simulink model "Reaction_Wheel_Model"  (R2025a)
settings: Solver=VariableStepAuto  StartTime=0.0  StopTime=120  RelTol=1e-3
values from neighbouring files (symbols this model uses):
  J = Jm + Jdisk    (= 1.0323014)    [Reaction_Wheel_Model_Variables.m]
  Js = 0.0022    [Reaction_Wheel_Model_Variables.m]
  K = 0.022    [Reaction_Wheel_Model_Variables.m]
  L = 580*10^-6    (= 0.00058)    [Reaction_Wheel_Model_Variables.m]
  R = 5.3    [Reaction_Wheel_Model_Variables.m]
libraries: simulink_extras x2
settings Model: Creator=Stefan1  LastModifiedBy=Stefan1

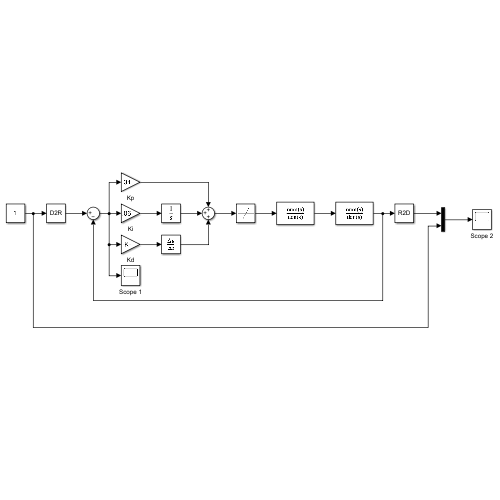
[thumbnail: Simulink's stored preview of the top-level diagram]
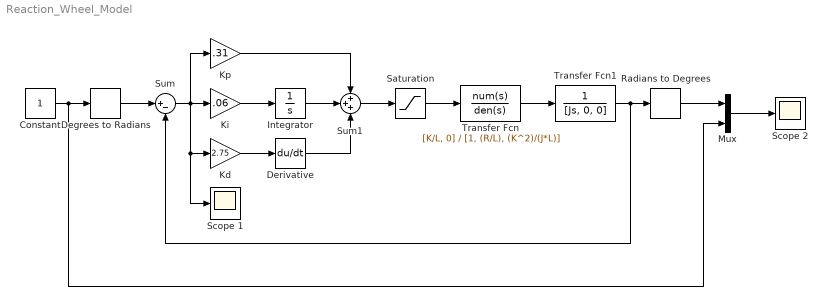
== system Reaction_Wheel_Model ==
  Constant : Constant
  Degrees to Radians : simulink_extras/Transformations/Degrees to Radians
  Derivative : Derivative
  Integrator : Integrator
  Kd : Gain  Gain=2.75
  Ki : Gain  Gain=.06
  Kp : Gain  Gain=.31
  Mux : Mux  Inputs=2
  Radians to Degrees : simulink_extras/Transformations/Radians to Degrees
  Saturation : Saturate  UpperLimit=12  LowerLimit=-12
  Scope 1 : Scope
      settings: ActiveDisplayYMinimum=-0.019743839684463423  ActiveDisplayYMaximum=0.022392181213908745
  Scope 2 : Scope
      settings: ActiveDisplayYMinimum=-29.385263692361058  ActiveDisplayYMaximum=20.546572996044425
  Sum : Sum  Inputs=|+-
  Sum1 : Sum  Inputs=+++
  Transfer Fcn : TransferFcn  Numerator=[K/L, 0]  Denominator=[1, (R/L), (K^2)/(J*L)]
  Transfer Fcn1 : TransferFcn  Denominator=[Js, 0, 0]
  wires:
  Kd/1 -> Derivative/1
  Ki/1 -> Integrator/1
  Integrator/1 -> Sum1/2
  Sum1/1 -> Saturation/1
  Constant/1 -> Mux/2, Degrees to Radians/1
  Degrees to Radians/1 -> Sum/1
  Sum/1 -> Scope 1/1, Kd/1, Kp/1, Ki/1
  Kp/1 -> Sum1/1
  Derivative/1 -> Sum1/3
  Saturation/1 -> Transfer Fcn/1
  Transfer Fcn/1 -> Transfer Fcn1/1
  Transfer Fcn1/1 -> Sum/2, Radians to Degrees/1
  Radians to Degrees/1 -> Mux/1
  Mux/1 -> Scope 2/1
